simulink model "Motor_Control"  (R2023b)
settings: Solver=VariableStepAuto  StartTime=0.0  StopTime=10.0  RelTol=1e-3
libraries: cstblocks x6
settings Model: Creator=dougl  LastModifiedBy=dougl

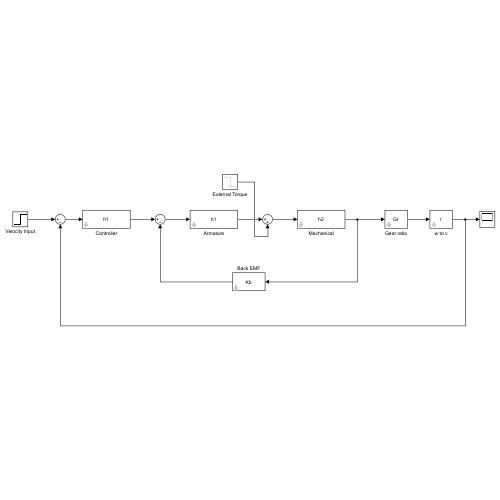
[thumbnail: Simulink's stored preview of the top-level diagram]
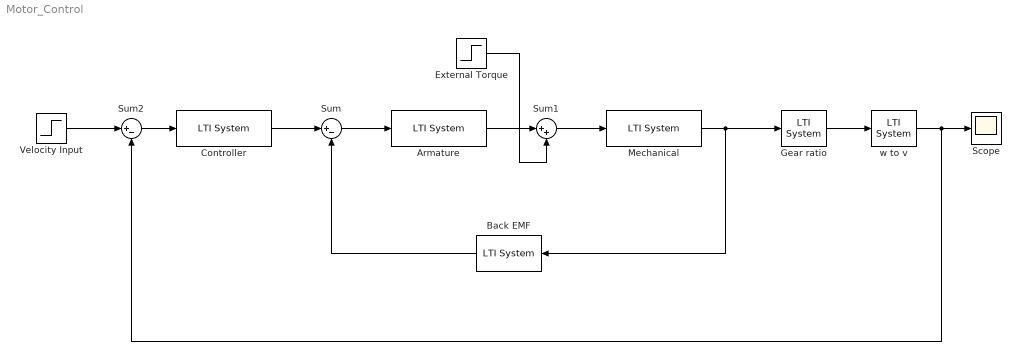
== system Motor_Control ==
  Armature : cstblocks/LTI System  sys=h1  IC=[]  PadeOrder=0
  Back EMF : cstblocks/LTI System  sys=Kb  IC=[]  PadeOrder=0
  Controller : cstblocks/LTI System  sys=h1  IC=[]  PadeOrder=0
  External Torque : Step  Time=5  After=-0.1  SampleTime=0
  Gear ratio : cstblocks/LTI System  sys=Gr  IC=[]  PadeOrder=0
  Mechanical : cstblocks/LTI System  sys=h2  IC=[]  PadeOrder=0
  Scope : Scope
  Sum : Sum  Inputs=|+-
  Sum1 : Sum  Inputs=|++
  Sum2 : Sum  Inputs=|+-
  Velocity Input : Step  Time=0.5  After=4  SampleTime=0
  w to v : cstblocks/LTI System  sys=r  IC=[]  PadeOrder=0
  wires:
  Sum/1 -> Armature/1
  Armature/1 -> Sum1/1
  Controller/1 -> Sum/1
  Sum1/1 -> Mechanical/1
  Mechanical/1 -> Gear ratio/1, Back EMF/1
  Back EMF/1 -> Sum/2
  Gear ratio/1 -> w to v/1
  External Torque/1 -> Sum1/2
  w to v/1 -> Sum2/2, Scope/1
  Sum2/1 -> Controller/1
  Velocity Input/1 -> Sum2/1
